simulink model "OFDM_Tx_Rx_Loopback"  (R2020a)
settings: Solver=FixedStepDiscrete  StartTime=0.0  StopTime=inf  RelTol=1e-3
InitFcn:
  | % Set parameters
  | fs = 200e3;
  | 
  | % Load all required variables
  | load('read_addr_data');
  | load('read_addr_cp');
  | load('read_addr_pream');
  | load('read_addr_rx');
  | load('pilot');
  | load('LTSfreq');
  | load('STSfreq');
  | load('LTSread');
  | load('STSread');
  | load('bpsk');
  | load('qpsk');
  | load('qam16');
values from neighbouring files (symbols this model uses):
  bpsk = [0 0 1 1 1 1 0 0 1 0 1 0 ... (48 elements, 48x1)]    [bpsk.mat]
  qam16 = [12 5 10 3 14 8 1 10 8 7 2 13 ... (48 elements, 48x1)]    [qam16.mat]
  qpsk = [1 2 1 2 2 2 3 1 1 3 1 0 ... (48 elements, 48x1)]    [qpsk.mat]
  STSfreq = [0 0 0 0 0 0 0 0 1 0 0 0 ... (64 elements, 1x64)]    [STSfreq.mat]
undefined symbols (not defined in the file or in its folder): data3, LTSfreq, LTSread, pilot, read_addr_cp, read_addr_data, read_addr_pream, read_addr_rx, STSread
libraries: hdlsllib x54, simulink x27, dsphdlxfrm x2, dsphdlsigops x1, dsphdlmathfun x1
(part 3 of 4)

== system OFDM_Tx_Rx_Loopback/OFDMRx/ChannelEstEq/DataArrange/SCReArrange/READ_CTRL ==
  In1 : Inport
  In2 : Inport  Port=2
  Constant : Constant  Value=0  OutDataTypeStr=fixdt(0,7,0)  SampleTime=1/fs
  Switch : Switch  Criteria=u2 ~= 0
  Out1 : Outport  VectorParamsAs1DForOutWhenUnconnected=off
  wires:
  Constant/1 -> Switch/3
  In2/1 -> Switch/2
  In1/1 -> Switch/1
  Switch/1 -> Out1/1

== system OFDM_Tx_Rx_Loopback/OFDMRx/Synchronisation/CoarseTiming/CoarseTimeStrobeGen/LocalSearchCounter ==
  note: Counter starts at 0
  note: Sample counter which is for local serach of X samples
      | after frame starting point. The counter resets
      | after X samples and is only initiated when the frame
      | detection pulse goes HIGH.
  packDetIn : Inport
  Compare To Constant : simulink/Logic and Bit Operations/Compare To Constant  relop===  const=19  OutDataTypeStr=boolean
  Constant : Constant  OutDataTypeStr=boolean  SampleTime=1/fs
  HDL Counter : hdlsllib/Sources/HDL Counter  CountType=Count limited  CountInit=0  CountStep=1  CountMax=19  CountFromType=Initial value  CountFrom=0  CountResetPort=on  CountLoadPort=off  CountEnbPort=on  CountDirPort=off  CountDataType=Unsigned  CountWordLen=8  CountFracLen=0  CountSampTime=1
  NOT : Logic  Operator=NOT  IconShape=distinctive  AllPortsSameDT=off  OutDataTypeStr=boolean
  RsingEdge : Subsystem
  Unit Delay Enabled Resettable Synchronous : hdlsllib/Discrete/Unit Delay Enabled Resettable Synchronous  InitialCondition=0.0  SampleTime=-1
      settings: SourceProductBaseCode=SL
  coutEnb : Outport  VectorParamsAs1DForOutWhenUnconnected=off
  countOut : Outport  Port=2  VectorParamsAs1DForOutWhenUnconnected=off
  wires:
  Unit Delay Enabled Resettable Synchronous/1 -> NOT/1, HDL Counter/2, coutEnb/1
  Compare To Constant/1 -> Unit Delay Enabled Resettable Synchronous/3
  Constant/1 -> Unit Delay Enabled Resettable Synchronous/1
  HDL Counter/1 -> Compare To Constant/1, countOut/1
  RsingEdge/1(Out1) -> Unit Delay Enabled Resettable Synchronous/2
  packDetIn/1 -> RsingEdge/1(In1)
  NOT/1 -> HDL Counter/1

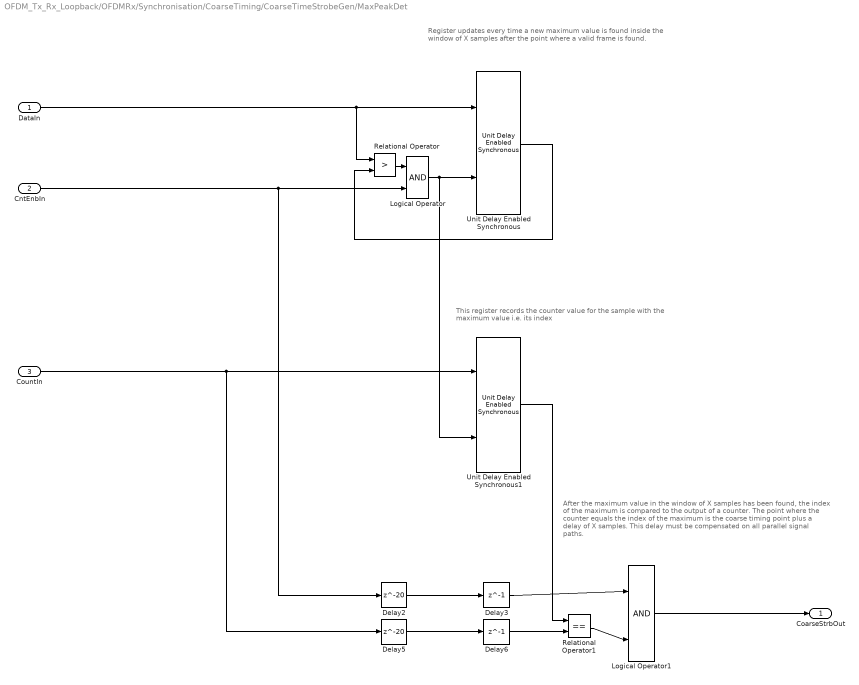
== system OFDM_Tx_Rx_Loopback/OFDMRx/Synchronisation/CoarseTiming/CoarseTimeStrobeGen/MaxPeakDet ==
  note: After the maximum value in the window of X samples has
      | been found, the index of the maximum is compared to the
      | output of a counter. The point where the counter equals the
      | index of the maximum is the coarse timing point plus a delay
      | of X samples. This delay must be compensated on all parallel
      | signal paths.
  note: This register records the counter value for the sample
      | with the maximum value i.e. its index
  note: Register updates every time a new maximum value is
      | found inside the window of X samples after the point where
      | a valid frame is found.
  DataIn : Inport
  CntEnbIn : Inport  Port=2
  CountIn : Inport  Port=3
  Delay2 : Delay  DelayLength=20
  Delay3 : Delay  DelayLength=1
  Delay5 : Delay  DelayLength=20
  Delay6 : Delay  DelayLength=1
  Logical Operator : Logic  IconShape=distinctive  AllPortsSameDT=off  OutDataTypeStr=boolean
  Logical Operator1 : Logic  IconShape=distinctive  AllPortsSameDT=off  OutDataTypeStr=boolean
  Relational Operator : RelationalOperator  Operator=>  OutDataTypeStr=boolean  RndMeth=Nearest
  Relational Operator1 : RelationalOperator  Operator===  OutDataTypeStr=boolean  RndMeth=Nearest
  Unit Delay Enabled Synchronous : hdlsllib/Discrete/Unit Delay Enabled Synchronous  InitialCondition=0.0  SampleTime=-1
      settings: SourceProductBaseCode=SL
  Unit Delay Enabled Synchronous1 : hdlsllib/Discrete/Unit Delay Enabled Synchronous  InitialCondition=0.0  SampleTime=-1
      settings: SourceProductBaseCode=SL
  CoarseStrbOut : Outport  VectorParamsAs1DForOutWhenUnconnected=off
  wires:
  Logical Operator1/1 -> CoarseStrbOut/1
  CountIn/1 -> Delay5/1, Unit Delay Enabled Synchronous1/1
  CntEnbIn/1 -> Delay2/1, Logical Operator/2
  Delay5/1 -> Delay6/1
  Unit Delay Enabled Synchronous/1 -> Relational Operator/2
  Unit Delay Enabled Synchronous1/1 -> Relational Operator1/1
  Relational Operator1/1 -> Logical Operator1/2
  Delay3/1 -> Logical Operator1/1
  Delay2/1 -> Delay3/1
  Relational Operator/1 -> Logical Operator/1
  DataIn/1 -> Unit Delay Enabled Synchronous/1, Relational Operator/1
  Logical Operator/1 -> Unit Delay Enabled Synchronous/2, Unit Delay Enabled Synchronous1/2
  Delay6/1 -> Relational Operator1/2

== system OFDM_Tx_Rx_Loopback/OFDMRx/Synchronisation/ControlSigGen/PreambleValidGen/RisingEdge ==
  ValidIn : Inport
  Delay : Delay  DelayLength=1
  Relational Operator : RelationalOperator  Operator=>  OutDataTypeStr=boolean  RndMeth=Nearest
  Out1 : Outport
  wires:
  Relational Operator/1 -> Out1/1
  Delay/1 -> Relational Operator/2
  ValidIn/1 -> Delay/1, Relational Operator/1

== system OFDM_Tx_Rx_Loopback/OFDMRx/Synchronisation/FineTimingSynch/MatchedFilter/Adder ==
  In1 : Inport
  In2 : Inport  Port=2
  Add : Sum  AccumDataTypeStr=fixdt(1,24,14)
  Delay3 : Delay  DelayLength=1
  Out1 : Outport  VectorParamsAs1DForOutWhenUnconnected=off
  wires:
  In2/1 -> Delay3/1
  In1/1 -> Add/1
  Add/1 -> Out1/1
  Delay3/1 -> Add/2

== system OFDM_Tx_Rx_Loopback/OFDMRx/Synchronisation/FineTimingSynch/MatchedFilter/Adder1 ==
  In1 : Inport
  In2 : Inport  Port=2
  Add : Sum  AccumDataTypeStr=fixdt(1,24,14)
  Delay3 : Delay  DelayLength=1
  Out1 : Outport  VectorParamsAs1DForOutWhenUnconnected=off
  wires:
  Delay3/1 -> Add/2
  Add/1 -> Out1/1
  In1/1 -> Add/1
  In2/1 -> Delay3/1

== system OFDM_Tx_Rx_Loopback/OFDMRx/Synchronisation/FineTimingSynch/MatchedFilter/Adder10 ==
  In1 : Inport
  In2 : Inport  Port=2
  Add : Sum  AccumDataTypeStr=fixdt(1,24,14)
  Delay3 : Delay  DelayLength=1
  Out1 : Outport  VectorParamsAs1DForOutWhenUnconnected=off
  wires:
  In2/1 -> Delay3/1
  In1/1 -> Add/1
  Add/1 -> Out1/1
  Delay3/1 -> Add/2

== system OFDM_Tx_Rx_Loopback/OFDMRx/Synchronisation/FineTimingSynch/MatchedFilter/Adder11 ==
  In1 : Inport
  In2 : Inport  Port=2
  Add : Sum  AccumDataTypeStr=fixdt(1,24,14)
  Delay3 : Delay  DelayLength=1
  Out1 : Outport  VectorParamsAs1DForOutWhenUnconnected=off
  wires:
  Delay3/1 -> Add/2
  Add/1 -> Out1/1
  In1/1 -> Add/1
  In2/1 -> Delay3/1

== system OFDM_Tx_Rx_Loopback/OFDMRx/Synchronisation/FineTimingSynch/MatchedFilter/Adder12 ==
  In1 : Inport
  In2 : Inport  Port=2
  Add : Sum  AccumDataTypeStr=fixdt(1,24,14)
  Delay3 : Delay  DelayLength=1
  Out1 : Outport  VectorParamsAs1DForOutWhenUnconnected=off
  wires:
  In2/1 -> Delay3/1
  In1/1 -> Add/1
  Add/1 -> Out1/1
  Delay3/1 -> Add/2

== system OFDM_Tx_Rx_Loopback/OFDMRx/Synchronisation/FineTimingSynch/MatchedFilter/Adder13 ==
  In1 : Inport
  In2 : Inport  Port=2
  Add : Sum  AccumDataTypeStr=fixdt(1,24,14)
  Delay3 : Delay  DelayLength=1
  Out1 : Outport  VectorParamsAs1DForOutWhenUnconnected=off
  wires:
  Delay3/1 -> Add/2
  Add/1 -> Out1/1
  In1/1 -> Add/1
  In2/1 -> Delay3/1

== system OFDM_Tx_Rx_Loopback/OFDMRx/Synchronisation/FineTimingSynch/MatchedFilter/Adder14 ==
  In1 : Inport
  In2 : Inport  Port=2
  Add : Sum  AccumDataTypeStr=fixdt(1,24,14)
  Delay3 : Delay  DelayLength=1
  Out1 : Outport  VectorParamsAs1DForOutWhenUnconnected=off
  wires:
  In2/1 -> Delay3/1
  In1/1 -> Add/1
  Add/1 -> Out1/1
  Delay3/1 -> Add/2

== system OFDM_Tx_Rx_Loopback/OFDMRx/Synchronisation/FineTimingSynch/MatchedFilter/Adder15 ==
  In1 : Inport
  In2 : Inport  Port=2
  Add : Sum  AccumDataTypeStr=fixdt(1,24,14)
  Delay3 : Delay  DelayLength=1
  Out1 : Outport  VectorParamsAs1DForOutWhenUnconnected=off
  wires:
  Delay3/1 -> Add/2
  Add/1 -> Out1/1
  In1/1 -> Add/1
  In2/1 -> Delay3/1

== system OFDM_Tx_Rx_Loopback/OFDMRx/Synchronisation/FineTimingSynch/MatchedFilter/Adder16 ==
  In1 : Inport
  In2 : Inport  Port=2
  Add : Sum  AccumDataTypeStr=fixdt(1,24,14)
  Delay3 : Delay  DelayLength=1
  Out1 : Outport  VectorParamsAs1DForOutWhenUnconnected=off
  wires:
  In2/1 -> Delay3/1
  In1/1 -> Add/1
  Add/1 -> Out1/1
  Delay3/1 -> Add/2

== system OFDM_Tx_Rx_Loopback/OFDMRx/Synchronisation/FineTimingSynch/MatchedFilter/Adder17 ==
  In1 : Inport
  In2 : Inport  Port=2
  Add : Sum  AccumDataTypeStr=fixdt(1,24,14)
  Delay3 : Delay  DelayLength=1
  Out1 : Outport  VectorParamsAs1DForOutWhenUnconnected=off
  wires:
  Delay3/1 -> Add/2
  Add/1 -> Out1/1
  In1/1 -> Add/1
  In2/1 -> Delay3/1

== system OFDM_Tx_Rx_Loopback/OFDMRx/Synchronisation/FineTimingSynch/MatchedFilter/Adder18 ==
  In1 : Inport
  In2 : Inport  Port=2
  Add : Sum  AccumDataTypeStr=fixdt(1,24,14)
  Delay3 : Delay  DelayLength=1
  Out1 : Outport  VectorParamsAs1DForOutWhenUnconnected=off
  wires:
  In2/1 -> Delay3/1
  In1/1 -> Add/1
  Add/1 -> Out1/1
  Delay3/1 -> Add/2

== system OFDM_Tx_Rx_Loopback/OFDMRx/Synchronisation/FineTimingSynch/MatchedFilter/Adder19 ==
  In1 : Inport
  In2 : Inport  Port=2
  Add : Sum  AccumDataTypeStr=fixdt(1,24,14)
  Delay3 : Delay  DelayLength=1
  Out1 : Outport  VectorParamsAs1DForOutWhenUnconnected=off
  wires:
  In2/1 -> Delay3/1
  In1/1 -> Add/1
  Add/1 -> Out1/1
  Delay3/1 -> Add/2

== system OFDM_Tx_Rx_Loopback/OFDMRx/Synchronisation/FineTimingSynch/MatchedFilter/Adder2 ==
  In1 : Inport
  In2 : Inport  Port=2
  Add : Sum  AccumDataTypeStr=fixdt(1,24,14)
  Delay3 : Delay  DelayLength=1
  Out1 : Outport  VectorParamsAs1DForOutWhenUnconnected=off
  wires:
  In2/1 -> Delay3/1
  In1/1 -> Add/1
  Add/1 -> Out1/1
  Delay3/1 -> Add/2

== system OFDM_Tx_Rx_Loopback/OFDMRx/Synchronisation/FineTimingSynch/MatchedFilter/Adder20 ==
  In1 : Inport
  In2 : Inport  Port=2
  Add : Sum  AccumDataTypeStr=fixdt(1,24,14)
  Delay3 : Delay  DelayLength=1
  Out1 : Outport  VectorParamsAs1DForOutWhenUnconnected=off
  wires:
  In2/1 -> Delay3/1
  In1/1 -> Add/1
  Add/1 -> Out1/1
  Delay3/1 -> Add/2

== system OFDM_Tx_Rx_Loopback/OFDMRx/Synchronisation/FineTimingSynch/MatchedFilter/Adder21 ==
  In1 : Inport
  In2 : Inport  Port=2
  Add : Sum  AccumDataTypeStr=fixdt(1,24,14)
  Delay3 : Delay  DelayLength=1
  Out1 : Outport  VectorParamsAs1DForOutWhenUnconnected=off
  wires:
  In2/1 -> Delay3/1
  In1/1 -> Add/1
  Add/1 -> Out1/1
  Delay3/1 -> Add/2

== system OFDM_Tx_Rx_Loopback/OFDMRx/Synchronisation/FineTimingSynch/MatchedFilter/Adder22 ==
  In1 : Inport
  In2 : Inport  Port=2
  Add : Sum  AccumDataTypeStr=fixdt(1,24,14)
  Delay3 : Delay  DelayLength=1
  Out1 : Outport  VectorParamsAs1DForOutWhenUnconnected=off
  wires:
  In2/1 -> Delay3/1
  In1/1 -> Add/1
  Add/1 -> Out1/1
  Delay3/1 -> Add/2

== system OFDM_Tx_Rx_Loopback/OFDMRx/Synchronisation/FineTimingSynch/MatchedFilter/Adder23 ==
  In1 : Inport
  In2 : Inport  Port=2
  Add : Sum  AccumDataTypeStr=fixdt(1,24,14)
  Delay3 : Delay  DelayLength=1
  Out1 : Outport  VectorParamsAs1DForOutWhenUnconnected=off
  wires:
  In2/1 -> Delay3/1
  In1/1 -> Add/1
  Add/1 -> Out1/1
  Delay3/1 -> Add/2

== system OFDM_Tx_Rx_Loopback/OFDMRx/Synchronisation/FineTimingSynch/MatchedFilter/Adder24 ==
  In1 : Inport
  In2 : Inport  Port=2
  Add : Sum  AccumDataTypeStr=fixdt(1,24,14)
  Delay3 : Delay  DelayLength=1
  Out1 : Outport  VectorParamsAs1DForOutWhenUnconnected=off
  wires:
  In2/1 -> Delay3/1
  In1/1 -> Add/1
  Add/1 -> Out1/1
  Delay3/1 -> Add/2

== system OFDM_Tx_Rx_Loopback/OFDMRx/Synchronisation/FineTimingSynch/MatchedFilter/Adder25 ==
  In1 : Inport
  In2 : Inport  Port=2
  Add : Sum  AccumDataTypeStr=fixdt(1,24,14)
  Delay3 : Delay  DelayLength=1
  Out1 : Outport  VectorParamsAs1DForOutWhenUnconnected=off
  wires:
  In2/1 -> Delay3/1
  In1/1 -> Add/1
  Add/1 -> Out1/1
  Delay3/1 -> Add/2

== system OFDM_Tx_Rx_Loopback/OFDMRx/Synchronisation/FineTimingSynch/MatchedFilter/Adder26 ==
  In1 : Inport
  In2 : Inport  Port=2
  Add : Sum  AccumDataTypeStr=fixdt(1,24,14)
  Delay3 : Delay  DelayLength=1
  Out1 : Outport  VectorParamsAs1DForOutWhenUnconnected=off
  wires:
  In2/1 -> Delay3/1
  In1/1 -> Add/1
  Add/1 -> Out1/1
  Delay3/1 -> Add/2

== system OFDM_Tx_Rx_Loopback/OFDMRx/Synchronisation/FineTimingSynch/MatchedFilter/Adder27 ==
  In1 : Inport
  In2 : Inport  Port=2
  Add : Sum  AccumDataTypeStr=fixdt(1,24,14)
  Delay3 : Delay  DelayLength=1
  Out1 : Outport  VectorParamsAs1DForOutWhenUnconnected=off
  wires:
  In2/1 -> Delay3/1
  In1/1 -> Add/1
  Add/1 -> Out1/1
  Delay3/1 -> Add/2

== system OFDM_Tx_Rx_Loopback/OFDMRx/Synchronisation/FineTimingSynch/MatchedFilter/Adder28 ==
  In1 : Inport
  In2 : Inport  Port=2
  Add : Sum
  Delay3 : Delay  DelayLength=1
  Out1 : Outport  VectorParamsAs1DForOutWhenUnconnected=off
  wires:
  In2/1 -> Delay3/1
  In1/1 -> Add/1
  Add/1 -> Out1/1
  Delay3/1 -> Add/2

== system OFDM_Tx_Rx_Loopback/OFDMRx/Synchronisation/FineTimingSynch/MatchedFilter/Adder29 ==
  In1 : Inport
  In2 : Inport  Port=2
  Add : Sum  AccumDataTypeStr=fixdt(1,24,14)
  Delay3 : Delay  DelayLength=1
  Out1 : Outport  VectorParamsAs1DForOutWhenUnconnected=off
  wires:
  In2/1 -> Delay3/1
  In1/1 -> Add/1
  Add/1 -> Out1/1
  Delay3/1 -> Add/2

== system OFDM_Tx_Rx_Loopback/OFDMRx/Synchronisation/FineTimingSynch/MatchedFilter/Adder3 ==
  In1 : Inport
  In2 : Inport  Port=2
  Add : Sum  AccumDataTypeStr=fixdt(1,24,14)
  Delay3 : Delay  DelayLength=1
  Out1 : Outport  VectorParamsAs1DForOutWhenUnconnected=off
  wires:
  Delay3/1 -> Add/2
  Add/1 -> Out1/1
  In1/1 -> Add/1
  In2/1 -> Delay3/1

== system OFDM_Tx_Rx_Loopback/OFDMRx/Synchronisation/FineTimingSynch/MatchedFilter/Adder30 ==
  In1 : Inport
  In2 : Inport  Port=2
  Add : Sum  AccumDataTypeStr=fixdt(1,24,14)
  Delay3 : Delay  DelayLength=1
  Out1 : Outport  VectorParamsAs1DForOutWhenUnconnected=off
  wires:
  In2/1 -> Delay3/1
  In1/1 -> Add/1
  Add/1 -> Out1/1
  Delay3/1 -> Add/2

== system OFDM_Tx_Rx_Loopback/OFDMRx/Synchronisation/FineTimingSynch/MatchedFilter/Adder31 ==
  In1 : Inport
  In2 : Inport  Port=2
  Add : Sum  AccumDataTypeStr=fixdt(1,24,14)
  Delay3 : Delay  DelayLength=1
  Out1 : Outport  VectorParamsAs1DForOutWhenUnconnected=off
  wires:
  In2/1 -> Delay3/1
  In1/1 -> Add/1
  Add/1 -> Out1/1
  Delay3/1 -> Add/2

== system OFDM_Tx_Rx_Loopback/OFDMRx/Synchronisation/FineTimingSynch/MatchedFilter/Adder32 ==
  In1 : Inport
  In2 : Inport  Port=2
  Add : Sum  AccumDataTypeStr=fixdt(1,24,14)
  Delay3 : Delay  DelayLength=1
  Out1 : Outport  VectorParamsAs1DForOutWhenUnconnected=off
  wires:
  In2/1 -> Delay3/1
  In1/1 -> Add/1
  Add/1 -> Out1/1
  Delay3/1 -> Add/2

== system OFDM_Tx_Rx_Loopback/OFDMRx/Synchronisation/FineTimingSynch/MatchedFilter/Adder33 ==
  In1 : Inport
  In2 : Inport  Port=2
  Add : Sum  AccumDataTypeStr=fixdt(1,24,14)
  Delay3 : Delay  DelayLength=1
  Out1 : Outport  VectorParamsAs1DForOutWhenUnconnected=off
  wires:
  In2/1 -> Delay3/1
  In1/1 -> Add/1
  Add/1 -> Out1/1
  Delay3/1 -> Add/2

== system OFDM_Tx_Rx_Loopback/OFDMRx/Synchronisation/FineTimingSynch/MatchedFilter/Adder34 ==
  In1 : Inport
  In2 : Inport  Port=2
  Add : Sum  AccumDataTypeStr=fixdt(1,24,14)
  Delay3 : Delay  DelayLength=1
  Out1 : Outport  VectorParamsAs1DForOutWhenUnconnected=off
  wires:
  In2/1 -> Delay3/1
  In1/1 -> Add/1
  Add/1 -> Out1/1
  Delay3/1 -> Add/2

== system OFDM_Tx_Rx_Loopback/OFDMRx/Synchronisation/FineTimingSynch/MatchedFilter/Adder35 ==
  In1 : Inport
  In2 : Inport  Port=2
  Add : Sum  AccumDataTypeStr=fixdt(1,24,14)
  Delay3 : Delay  DelayLength=1
  Out1 : Outport  VectorParamsAs1DForOutWhenUnconnected=off
  wires:
  In2/1 -> Delay3/1
  In1/1 -> Add/1
  Add/1 -> Out1/1
  Delay3/1 -> Add/2

== system OFDM_Tx_Rx_Loopback/OFDMRx/Synchronisation/FineTimingSynch/MatchedFilter/Adder36 ==
  In1 : Inport
  In2 : Inport  Port=2
  Add : Sum  AccumDataTypeStr=fixdt(1,24,14)
  Delay3 : Delay  DelayLength=1
  Out1 : Outport  VectorParamsAs1DForOutWhenUnconnected=off
  wires:
  In2/1 -> Delay3/1
  In1/1 -> Add/1
  Add/1 -> Out1/1
  Delay3/1 -> Add/2

== system OFDM_Tx_Rx_Loopback/OFDMRx/Synchronisation/FineTimingSynch/MatchedFilter/Adder37 ==
  In1 : Inport
  In2 : Inport  Port=2
  Add : Sum  AccumDataTypeStr=fixdt(1,24,14)
  Delay3 : Delay  DelayLength=1
  Out1 : Outport  VectorParamsAs1DForOutWhenUnconnected=off
  wires:
  In2/1 -> Delay3/1
  In1/1 -> Add/1
  Add/1 -> Out1/1
  Delay3/1 -> Add/2

== system OFDM_Tx_Rx_Loopback/OFDMRx/Synchronisation/FineTimingSynch/MatchedFilter/Adder38 ==
  In1 : Inport
  In2 : Inport  Port=2
  Add : Sum  AccumDataTypeStr=fixdt(1,24,14)
  Delay3 : Delay  DelayLength=1
  Out1 : Outport  VectorParamsAs1DForOutWhenUnconnected=off
  wires:
  In2/1 -> Delay3/1
  In1/1 -> Add/1
  Add/1 -> Out1/1
  Delay3/1 -> Add/2

== system OFDM_Tx_Rx_Loopback/OFDMRx/Synchronisation/FineTimingSynch/MatchedFilter/Adder39 ==
  In1 : Inport
  In2 : Inport  Port=2
  Add : Sum  AccumDataTypeStr=fixdt(1,24,14)
  Delay3 : Delay  DelayLength=1
  Out1 : Outport  VectorParamsAs1DForOutWhenUnconnected=off
  wires:
  In2/1 -> Delay3/1
  In1/1 -> Add/1
  Add/1 -> Out1/1
  Delay3/1 -> Add/2

== system OFDM_Tx_Rx_Loopback/OFDMRx/Synchronisation/FineTimingSynch/MatchedFilter/Adder4 ==
  In1 : Inport
  In2 : Inport  Port=2
  Add : Sum  AccumDataTypeStr=fixdt(1,24,14)
  Delay3 : Delay  DelayLength=1
  Out1 : Outport  VectorParamsAs1DForOutWhenUnconnected=off
  wires:
  In2/1 -> Delay3/1
  In1/1 -> Add/1
  Add/1 -> Out1/1
  Delay3/1 -> Add/2

== system OFDM_Tx_Rx_Loopback/OFDMRx/Synchronisation/FineTimingSynch/MatchedFilter/Adder40 ==
  In1 : Inport
  In2 : Inport  Port=2
  Add : Sum  AccumDataTypeStr=fixdt(1,24,14)
  Delay3 : Delay  DelayLength=1
  Out1 : Outport  VectorParamsAs1DForOutWhenUnconnected=off
  wires:
  In2/1 -> Delay3/1
  In1/1 -> Add/1
  Add/1 -> Out1/1
  Delay3/1 -> Add/2

== system OFDM_Tx_Rx_Loopback/OFDMRx/Synchronisation/FineTimingSynch/MatchedFilter/Adder41 ==
  In1 : Inport
  In2 : Inport  Port=2
  Add : Sum  AccumDataTypeStr=fixdt(1,24,14)
  Delay3 : Delay  DelayLength=1
  Out1 : Outport  VectorParamsAs1DForOutWhenUnconnected=off
  wires:
  In2/1 -> Delay3/1
  In1/1 -> Add/1
  Add/1 -> Out1/1
  Delay3/1 -> Add/2

== system OFDM_Tx_Rx_Loopback/OFDMRx/Synchronisation/FineTimingSynch/MatchedFilter/Adder42 ==
  In1 : Inport
  In2 : Inport  Port=2
  Add : Sum  AccumDataTypeStr=fixdt(1,24,14)
  Delay3 : Delay  DelayLength=1
  Out1 : Outport  VectorParamsAs1DForOutWhenUnconnected=off
  wires:
  In2/1 -> Delay3/1
  In1/1 -> Add/1
  Add/1 -> Out1/1
  Delay3/1 -> Add/2

== system OFDM_Tx_Rx_Loopback/OFDMRx/Synchronisation/FineTimingSynch/MatchedFilter/Adder43 ==
  In1 : Inport
  In2 : Inport  Port=2
  Add : Sum  AccumDataTypeStr=fixdt(1,24,14)
  Delay3 : Delay  DelayLength=1
  Out1 : Outport  VectorParamsAs1DForOutWhenUnconnected=off
  wires:
  In2/1 -> Delay3/1
  In1/1 -> Add/1
  Add/1 -> Out1/1
  Delay3/1 -> Add/2

== system OFDM_Tx_Rx_Loopback/OFDMRx/Synchronisation/FineTimingSynch/MatchedFilter/Adder44 ==
  In1 : Inport
  In2 : Inport  Port=2
  Add : Sum  AccumDataTypeStr=fixdt(1,24,14)
  Delay3 : Delay  DelayLength=1
  Out1 : Outport  VectorParamsAs1DForOutWhenUnconnected=off
  wires:
  In2/1 -> Delay3/1
  In1/1 -> Add/1
  Add/1 -> Out1/1
  Delay3/1 -> Add/2

== system OFDM_Tx_Rx_Loopback/OFDMRx/Synchronisation/FineTimingSynch/MatchedFilter/Adder45 ==
  In1 : Inport
  In2 : Inport  Port=2
  Add : Sum  AccumDataTypeStr=fixdt(1,24,14)
  Delay3 : Delay  DelayLength=1
  Out1 : Outport  VectorParamsAs1DForOutWhenUnconnected=off
  wires:
  In2/1 -> Delay3/1
  In1/1 -> Add/1
  Add/1 -> Out1/1
  Delay3/1 -> Add/2

== system OFDM_Tx_Rx_Loopback/OFDMRx/Synchronisation/FineTimingSynch/MatchedFilter/Adder46 ==
  In1 : Inport
  In2 : Inport  Port=2
  Add : Sum  AccumDataTypeStr=fixdt(1,24,14)
  Delay3 : Delay  DelayLength=1
  Out1 : Outport  VectorParamsAs1DForOutWhenUnconnected=off
  wires:
  In2/1 -> Delay3/1
  In1/1 -> Add/1
  Add/1 -> Out1/1
  Delay3/1 -> Add/2

== system OFDM_Tx_Rx_Loopback/OFDMRx/Synchronisation/FineTimingSynch/MatchedFilter/Adder47 ==
  In1 : Inport
  In2 : Inport  Port=2
  Add : Sum  AccumDataTypeStr=fixdt(1,24,14)
  Delay3 : Delay  DelayLength=1
  Out1 : Outport  VectorParamsAs1DForOutWhenUnconnected=off
  wires:
  In2/1 -> Delay3/1
  In1/1 -> Add/1
  Add/1 -> Out1/1
  Delay3/1 -> Add/2

== system OFDM_Tx_Rx_Loopback/OFDMRx/Synchronisation/FineTimingSynch/MatchedFilter/Adder48 ==
  In1 : Inport
  In2 : Inport  Port=2
  Add : Sum  AccumDataTypeStr=fixdt(1,24,14)
  Delay3 : Delay  DelayLength=1
  Out1 : Outport  VectorParamsAs1DForOutWhenUnconnected=off
  wires:
  In2/1 -> Delay3/1
  In1/1 -> Add/1
  Add/1 -> Out1/1
  Delay3/1 -> Add/2

== system OFDM_Tx_Rx_Loopback/OFDMRx/Synchronisation/FineTimingSynch/MatchedFilter/Adder49 ==
  In1 : Inport
  In2 : Inport  Port=2
  Add : Sum  AccumDataTypeStr=fixdt(1,24,14)
  Delay3 : Delay  DelayLength=1
  Out1 : Outport  VectorParamsAs1DForOutWhenUnconnected=off
  wires:
  In2/1 -> Delay3/1
  In1/1 -> Add/1
  Add/1 -> Out1/1
  Delay3/1 -> Add/2

== system OFDM_Tx_Rx_Loopback/OFDMRx/Synchronisation/FineTimingSynch/MatchedFilter/Adder5 ==
  In1 : Inport
  In2 : Inport  Port=2
  Add : Sum  AccumDataTypeStr=fixdt(1,24,14)
  Delay3 : Delay  DelayLength=1
  Out1 : Outport  VectorParamsAs1DForOutWhenUnconnected=off
  wires:
  Delay3/1 -> Add/2
  Add/1 -> Out1/1
  In1/1 -> Add/1
  In2/1 -> Delay3/1

== system OFDM_Tx_Rx_Loopback/OFDMRx/Synchronisation/FineTimingSynch/MatchedFilter/Adder50 ==
  In1 : Inport
  In2 : Inport  Port=2
  Add : Sum  AccumDataTypeStr=fixdt(1,24,14)
  Delay3 : Delay  DelayLength=1
  Out1 : Outport  VectorParamsAs1DForOutWhenUnconnected=off
  wires:
  In2/1 -> Delay3/1
  In1/1 -> Add/1
  Add/1 -> Out1/1
  Delay3/1 -> Add/2

== system OFDM_Tx_Rx_Loopback/OFDMRx/Synchronisation/FineTimingSynch/MatchedFilter/Adder51 ==
  In1 : Inport
  In2 : Inport  Port=2
  Add : Sum  AccumDataTypeStr=fixdt(1,24,14)
  Delay3 : Delay  DelayLength=1
  Out1 : Outport  VectorParamsAs1DForOutWhenUnconnected=off
  wires:
  In2/1 -> Delay3/1
  In1/1 -> Add/1
  Add/1 -> Out1/1
  Delay3/1 -> Add/2

== system OFDM_Tx_Rx_Loopback/OFDMRx/Synchronisation/FineTimingSynch/MatchedFilter/Adder52 ==
  In1 : Inport
  In2 : Inport  Port=2
  Add : Sum  AccumDataTypeStr=fixdt(1,24,14)
  Delay3 : Delay  DelayLength=1
  Out1 : Outport  VectorParamsAs1DForOutWhenUnconnected=off
  wires:
  In2/1 -> Delay3/1
  In1/1 -> Add/1
  Add/1 -> Out1/1
  Delay3/1 -> Add/2

== system OFDM_Tx_Rx_Loopback/OFDMRx/Synchronisation/FineTimingSynch/MatchedFilter/Adder53 ==
  In1 : Inport
  In2 : Inport  Port=2
  Add : Sum  AccumDataTypeStr=fixdt(1,24,14)
  Delay3 : Delay  DelayLength=1
  Out1 : Outport  VectorParamsAs1DForOutWhenUnconnected=off
  wires:
  In2/1 -> Delay3/1
  In1/1 -> Add/1
  Add/1 -> Out1/1
  Delay3/1 -> Add/2

== system OFDM_Tx_Rx_Loopback/OFDMRx/Synchronisation/FineTimingSynch/MatchedFilter/Adder54 ==
  In1 : Inport
  In2 : Inport  Port=2
  Add : Sum  AccumDataTypeStr=fixdt(1,24,14)
  Delay3 : Delay  DelayLength=1
  Out1 : Outport  VectorParamsAs1DForOutWhenUnconnected=off
  wires:
  In2/1 -> Delay3/1
  In1/1 -> Add/1
  Add/1 -> Out1/1
  Delay3/1 -> Add/2

== system OFDM_Tx_Rx_Loopback/OFDMRx/Synchronisation/FineTimingSynch/MatchedFilter/Adder55 ==
  In1 : Inport
  In2 : Inport  Port=2
  Add : Sum  AccumDataTypeStr=fixdt(1,24,14)
  Delay3 : Delay  DelayLength=1
  Out1 : Outport  VectorParamsAs1DForOutWhenUnconnected=off
  wires:
  In2/1 -> Delay3/1
  In1/1 -> Add/1
  Add/1 -> Out1/1
  Delay3/1 -> Add/2

== system OFDM_Tx_Rx_Loopback/OFDMRx/Synchronisation/FineTimingSynch/MatchedFilter/Adder56 ==
  In1 : Inport
  In2 : Inport  Port=2
  Add : Sum  AccumDataTypeStr=fixdt(1,24,14)
  Delay3 : Delay  DelayLength=1
  Out1 : Outport  VectorParamsAs1DForOutWhenUnconnected=off
  wires:
  In2/1 -> Delay3/1
  In1/1 -> Add/1
  Add/1 -> Out1/1
  Delay3/1 -> Add/2

== system OFDM_Tx_Rx_Loopback/OFDMRx/Synchronisation/FineTimingSynch/MatchedFilter/Adder57 ==
  In1 : Inport
  In2 : Inport  Port=2
  Add : Sum  AccumDataTypeStr=fixdt(1,24,14)
  Delay3 : Delay  DelayLength=1
  Out1 : Outport  VectorParamsAs1DForOutWhenUnconnected=off
  wires:
  In2/1 -> Delay3/1
  In1/1 -> Add/1
  Add/1 -> Out1/1
  Delay3/1 -> Add/2

== system OFDM_Tx_Rx_Loopback/OFDMRx/Synchronisation/FineTimingSynch/MatchedFilter/Adder58 ==
  In1 : Inport
  In2 : Inport  Port=2
  Add : Sum  AccumDataTypeStr=fixdt(1,24,14)
  Delay3 : Delay  DelayLength=1
  Out1 : Outport  VectorParamsAs1DForOutWhenUnconnected=off
  wires:
  In2/1 -> Delay3/1
  In1/1 -> Add/1
  Add/1 -> Out1/1
  Delay3/1 -> Add/2

== system OFDM_Tx_Rx_Loopback/OFDMRx/Synchronisation/FineTimingSynch/MatchedFilter/Adder59 ==
  In1 : Inport
  In2 : Inport  Port=2
  Add : Sum  AccumDataTypeStr=fixdt(1,24,14)
  Delay3 : Delay  DelayLength=1
  Out1 : Outport  VectorParamsAs1DForOutWhenUnconnected=off
  wires:
  In2/1 -> Delay3/1
  In1/1 -> Add/1
  Add/1 -> Out1/1
  Delay3/1 -> Add/2

== system OFDM_Tx_Rx_Loopback/OFDMRx/Synchronisation/FineTimingSynch/MatchedFilter/Adder6 ==
  In1 : Inport
  In2 : Inport  Port=2
  Add : Sum  AccumDataTypeStr=fixdt(1,24,14)
  Delay3 : Delay  DelayLength=1
  Out1 : Outport  VectorParamsAs1DForOutWhenUnconnected=off
  wires:
  In2/1 -> Delay3/1
  In1/1 -> Add/1
  Add/1 -> Out1/1
  Delay3/1 -> Add/2

== system OFDM_Tx_Rx_Loopback/OFDMRx/Synchronisation/FineTimingSynch/MatchedFilter/Adder60 ==
  In1 : Inport
  In2 : Inport  Port=2
  Add : Sum  AccumDataTypeStr=fixdt(1,24,14)
  Delay3 : Delay  DelayLength=1
  Out1 : Outport  VectorParamsAs1DForOutWhenUnconnected=off
  wires:
  In2/1 -> Delay3/1
  In1/1 -> Add/1
  Add/1 -> Out1/1
  Delay3/1 -> Add/2

== system OFDM_Tx_Rx_Loopback/OFDMRx/Synchronisation/FineTimingSynch/MatchedFilter/Adder61 ==
  In1 : Inport
  In2 : Inport  Port=2
  Add : Sum  AccumDataTypeStr=fixdt(1,24,14)
  Delay3 : Delay  DelayLength=1
  Out1 : Outport  VectorParamsAs1DForOutWhenUnconnected=off
  wires:
  In2/1 -> Delay3/1
  In1/1 -> Add/1
  Add/1 -> Out1/1
  Delay3/1 -> Add/2

== system OFDM_Tx_Rx_Loopback/OFDMRx/Synchronisation/FineTimingSynch/MatchedFilter/Adder62 ==
  In1 : Inport
  In2 : Inport  Port=2
  Add : Sum  AccumDataTypeStr=fixdt(1,24,14)
  Delay3 : Delay  DelayLength=1
  Out1 : Outport  VectorParamsAs1DForOutWhenUnconnected=off
  wires:
  In2/1 -> Delay3/1
  In1/1 -> Add/1
  Add/1 -> Out1/1
  Delay3/1 -> Add/2

== system OFDM_Tx_Rx_Loopback/OFDMRx/Synchronisation/FineTimingSynch/MatchedFilter/Adder7 ==
  In1 : Inport
  In2 : Inport  Port=2
  Add : Sum  AccumDataTypeStr=fixdt(1,24,14)
  Delay3 : Delay  DelayLength=1
  Out1 : Outport  VectorParamsAs1DForOutWhenUnconnected=off
  wires:
  Delay3/1 -> Add/2
  Add/1 -> Out1/1
  In1/1 -> Add/1
  In2/1 -> Delay3/1

== system OFDM_Tx_Rx_Loopback/OFDMRx/Synchronisation/FineTimingSynch/MatchedFilter/Adder8 ==
  In1 : Inport
  In2 : Inport  Port=2
  Add : Sum  AccumDataTypeStr=fixdt(1,24,14)
  Delay3 : Delay  DelayLength=1
  Out1 : Outport  VectorParamsAs1DForOutWhenUnconnected=off
  wires:
  In2/1 -> Delay3/1
  In1/1 -> Add/1
  Add/1 -> Out1/1
  Delay3/1 -> Add/2

== system OFDM_Tx_Rx_Loopback/OFDMRx/Synchronisation/FineTimingSynch/MatchedFilter/Adder9 ==
  In1 : Inport
  In2 : Inport  Port=2
  Add : Sum  AccumDataTypeStr=fixdt(1,24,14)
  Delay3 : Delay  DelayLength=1
  Out1 : Outport  VectorParamsAs1DForOutWhenUnconnected=off
  wires:
  Delay3/1 -> Add/2
  Add/1 -> Out1/1
  In1/1 -> Add/1
  In2/1 -> Delay3/1

== system OFDM_Tx_Rx_Loopback/OFDMRx/Synchronisation/FineTimingSynch/MatchedFilter/Subsystem ==
  MatchedIn : Inport
  Add : Sum  OutDataTypeStr=fixdt(1,18,14)
  Add1 : Sum  Inputs=+-  OutDataTypeStr=fixdt(1,18,14)
  Complex to Real-Imag : ComplexToRealImag
  Real-Imag to Complex : RealImagToComplex
  Unary Minus : UnaryMinus
  Out1 : Outport
  wires:
  Real-Imag to Complex/1 -> Out1/1
  MatchedIn/1 -> Complex to Real-Imag/1
  Add1/1 -> Real-Imag to Complex/1
  Complex to Real-Imag/2 -> Add/2, Add1/1
  Complex to Real-Imag/1 -> Add/1, Add1/2
  Add/1 -> Unary Minus/1
  Unary Minus/1 -> Real-Imag to Complex/2

== system OFDM_Tx_Rx_Loopback/OFDMRx/Synchronisation/FineTimingSynch/MatchedFilter/Subsystem1 ==
  MatchedIn : Inport
  Add : Sum  OutDataTypeStr=fixdt(1,18,14)
  Add1 : Sum  Inputs=+-  OutDataTypeStr=fixdt(1,18,14)
  Complex to Real-Imag : ComplexToRealImag
  Real-Imag to Complex : RealImagToComplex
  Out1 : Outport
  wires:
  Complex to Real-Imag/2 -> Add1/1, Add/2
  Add/1 -> Real-Imag to Complex/1
  Add1/1 -> Real-Imag to Complex/2
  Complex to Real-Imag/1 -> Add1/2, Add/1
  MatchedIn/1 -> Complex to Real-Imag/1
  Real-Imag to Complex/1 -> Out1/1

== system OFDM_Tx_Rx_Loopback/OFDMRx/Synchronisation/FineTimingSynch/MatchedFilter/Subsystem10 ==
  MatchedIn : Inport
  Add : Sum  OutDataTypeStr=fixdt(1,18,14)
  Add1 : Sum  Inputs=+-  OutDataTypeStr=fixdt(1,18,14)
  Complex to Real-Imag : ComplexToRealImag
  Real-Imag to Complex : RealImagToComplex
  Unary Minus : UnaryMinus
  Out1 : Outport
  wires:
  Unary Minus/1 -> Real-Imag to Complex/2
  Add/1 -> Unary Minus/1
  Complex to Real-Imag/1 -> Add1/2, Add/1
  Complex to Real-Imag/2 -> Add1/1, Add/2
  Add1/1 -> Real-Imag to Complex/1
  MatchedIn/1 -> Complex to Real-Imag/1
  Real-Imag to Complex/1 -> Out1/1

== system OFDM_Tx_Rx_Loopback/OFDMRx/Synchronisation/FineTimingSynch/MatchedFilter/Subsystem11 ==
  MatchedIn : Inport
  Add : Sum  OutDataTypeStr=fixdt(1,18,14)
  Add1 : Sum  Inputs=+-  OutDataTypeStr=fixdt(1,18,14)
  Complex to Real-Imag : ComplexToRealImag
  Real-Imag to Complex : RealImagToComplex
  Out1 : Outport
  wires:
  Real-Imag to Complex/1 -> Out1/1
  MatchedIn/1 -> Complex to Real-Imag/1
  Complex to Real-Imag/1 -> Add/1, Add1/2
  Add1/1 -> Real-Imag to Complex/2
  Add/1 -> Real-Imag to Complex/1
  Complex to Real-Imag/2 -> Add/2, Add1/1

== system OFDM_Tx_Rx_Loopback/OFDMRx/Synchronisation/FineTimingSynch/MatchedFilter/Subsystem12 ==
  MatchedIn : Inport
  Add : Sum  OutDataTypeStr=fixdt(1,18,14)
  Add1 : Sum  Inputs=+-  OutDataTypeStr=fixdt(1,18,14)
  Complex to Real-Imag : ComplexToRealImag
  Real-Imag to Complex : RealImagToComplex
  Out1 : Outport
  wires:
  Real-Imag to Complex/1 -> Out1/1
  MatchedIn/1 -> Complex to Real-Imag/1
  Complex to Real-Imag/1 -> Add/1, Add1/2
  Add1/1 -> Real-Imag to Complex/2
  Add/1 -> Real-Imag to Complex/1
  Complex to Real-Imag/2 -> Add/2, Add1/1

== system OFDM_Tx_Rx_Loopback/OFDMRx/Synchronisation/FineTimingSynch/MatchedFilter/Subsystem13 ==
  MatchedIn : Inport
  Add : Sum  OutDataTypeStr=fixdt(1,18,14)
  Add1 : Sum  Inputs=+-  OutDataTypeStr=fixdt(1,18,14)
  Complex to Real-Imag : ComplexToRealImag
  Real-Imag to Complex : RealImagToComplex
  Unary Minus : UnaryMinus
  Out1 : Outport
  wires:
  Complex to Real-Imag/2 -> Add1/2, Add/2
  Add/1 -> Unary Minus/1
  Add1/1 -> Real-Imag to Complex/2
  Complex to Real-Imag/1 -> Add1/1, Add/1
  MatchedIn/1 -> Complex to Real-Imag/1
  Real-Imag to Complex/1 -> Out1/1
  Unary Minus/1 -> Real-Imag to Complex/1

== system OFDM_Tx_Rx_Loopback/OFDMRx/Synchronisation/FineTimingSynch/MatchedFilter/Subsystem14 ==
  MatchedIn : Inport
  Add : Sum  OutDataTypeStr=fixdt(1,18,14)
  Add1 : Sum  Inputs=+-  OutDataTypeStr=fixdt(1,18,14)
  Complex to Real-Imag : ComplexToRealImag
  Real-Imag to Complex : RealImagToComplex
  Out1 : Outport
  wires:
  Real-Imag to Complex/1 -> Out1/1
  MatchedIn/1 -> Complex to Real-Imag/1
  Complex to Real-Imag/1 -> Add/1, Add1/2
  Add1/1 -> Real-Imag to Complex/2
  Add/1 -> Real-Imag to Complex/1
  Complex to Real-Imag/2 -> Add/2, Add1/1

== system OFDM_Tx_Rx_Loopback/OFDMRx/Synchronisation/FineTimingSynch/MatchedFilter/Subsystem15 ==
  MatchedIn : Inport
  Add : Sum  OutDataTypeStr=fixdt(1,18,14)
  Add1 : Sum  Inputs=+-  OutDataTypeStr=fixdt(1,18,14)
  Complex to Real-Imag : ComplexToRealImag
  Real-Imag to Complex : RealImagToComplex
  Out1 : Outport
  wires:
  Real-Imag to Complex/1 -> Out1/1
  MatchedIn/1 -> Complex to Real-Imag/1
  Complex to Real-Imag/1 -> Add/1, Add1/2
  Add1/1 -> Real-Imag to Complex/2
  Add/1 -> Real-Imag to Complex/1
  Complex to Real-Imag/2 -> Add/2, Add1/1

== system OFDM_Tx_Rx_Loopback/OFDMRx/Synchronisation/FineTimingSynch/MatchedFilter/Subsystem16 ==
  MatchedIn : Inport
  Add : Sum  OutDataTypeStr=fixdt(1,18,14)
  Add1 : Sum  Inputs=+-  OutDataTypeStr=fixdt(1,18,14)
  Complex to Real-Imag : ComplexToRealImag
  Real-Imag to Complex : RealImagToComplex
  Out1 : Outport
  wires:
  Add/1 -> Real-Imag to Complex/2
  Add1/1 -> Real-Imag to Complex/1
  Complex to Real-Imag/2 -> Add/2, Add1/2
  Complex to Real-Imag/1 -> Add/1, Add1/1
  MatchedIn/1 -> Complex to Real-Imag/1
  Real-Imag to Complex/1 -> Out1/1

== system OFDM_Tx_Rx_Loopback/OFDMRx/Synchronisation/FineTimingSynch/MatchedFilter/Subsystem17 ==
  MatchedIn : Inport
  Add : Sum  OutDataTypeStr=fixdt(1,18,14)
  Add1 : Sum  Inputs=+-  OutDataTypeStr=fixdt(1,18,14)
  Complex to Real-Imag : ComplexToRealImag
  Real-Imag to Complex : RealImagToComplex
  Unary Minus : UnaryMinus
  Out1 : Outport
  wires:
  Unary Minus/1 -> Real-Imag to Complex/1
  Real-Imag to Complex/1 -> Out1/1
  MatchedIn/1 -> Complex to Real-Imag/1
  Complex to Real-Imag/1 -> Add/1, Add1/1
  Add1/1 -> Real-Imag to Complex/2
  Add/1 -> Unary Minus/1
  Complex to Real-Imag/2 -> Add/2, Add1/2

== system OFDM_Tx_Rx_Loopback/OFDMRx/Synchronisation/FineTimingSynch/MatchedFilter/Subsystem18 ==
  MatchedIn : Inport
  Add : Sum  OutDataTypeStr=fixdt(1,18,14)
  Add1 : Sum  Inputs=+-  OutDataTypeStr=fixdt(1,18,14)
  Complex to Real-Imag : ComplexToRealImag
  Real-Imag to Complex : RealImagToComplex
  Unary Minus : UnaryMinus
  Out1 : Outport
  wires:
  Unary Minus/1 -> Real-Imag to Complex/1
  Real-Imag to Complex/1 -> Out1/1
  MatchedIn/1 -> Complex to Real-Imag/1
  Complex to Real-Imag/1 -> Add/1, Add1/1
  Add1/1 -> Real-Imag to Complex/2
  Add/1 -> Unary Minus/1
  Complex to Real-Imag/2 -> Add/2, Add1/2

== system OFDM_Tx_Rx_Loopback/OFDMRx/Synchronisation/FineTimingSynch/MatchedFilter/Subsystem19 ==
  MatchedIn : Inport
  Add : Sum  OutDataTypeStr=fixdt(1,18,14)
  Add1 : Sum  Inputs=+-  OutDataTypeStr=fixdt(1,18,14)
  Complex to Real-Imag : ComplexToRealImag
  Real-Imag to Complex : RealImagToComplex
  Out1 : Outport
  wires:
  Add/1 -> Real-Imag to Complex/2
  Add1/1 -> Real-Imag to Complex/1
  Complex to Real-Imag/2 -> Add/2, Add1/2
  Complex to Real-Imag/1 -> Add/1, Add1/1
  MatchedIn/1 -> Complex to Real-Imag/1
  Real-Imag to Complex/1 -> Out1/1

== system OFDM_Tx_Rx_Loopback/OFDMRx/Synchronisation/FineTimingSynch/MatchedFilter/Subsystem2 ==
  MatchedIn : Inport
  Add : Sum  OutDataTypeStr=fixdt(1,18,14)
  Add1 : Sum  Inputs=+-  OutDataTypeStr=fixdt(1,18,14)
  Complex to Real-Imag : ComplexToRealImag
  Real-Imag to Complex : RealImagToComplex
  Out1 : Outport
  wires:
  Real-Imag to Complex/1 -> Out1/1
  MatchedIn/1 -> Complex to Real-Imag/1
  Complex to Real-Imag/1 -> Add1/1, Add/1
  Complex to Real-Imag/2 -> Add1/2, Add/2
  Add1/1 -> Real-Imag to Complex/1
  Add/1 -> Real-Imag to Complex/2

== system OFDM_Tx_Rx_Loopback/OFDMRx/Synchronisation/FineTimingSynch/MatchedFilter/Subsystem20 ==
  MatchedIn : Inport
  Add : Sum  OutDataTypeStr=fixdt(1,18,14)
  Add1 : Sum  Inputs=+-  OutDataTypeStr=fixdt(1,18,14)
  Complex to Real-Imag : ComplexToRealImag
  Real-Imag to Complex : RealImagToComplex
  Out1 : Outport
  wires:
  Add/1 -> Real-Imag to Complex/2
  Add1/1 -> Real-Imag to Complex/1
  Complex to Real-Imag/2 -> Add/2, Add1/2
  Complex to Real-Imag/1 -> Add/1, Add1/1
  MatchedIn/1 -> Complex to Real-Imag/1
  Real-Imag to Complex/1 -> Out1/1

== system OFDM_Tx_Rx_Loopback/OFDMRx/Synchronisation/FineTimingSynch/MatchedFilter/Subsystem21 ==
  MatchedIn : Inport
  Add : Sum  OutDataTypeStr=fixdt(1,18,14)
  Add1 : Sum  Inputs=+-  OutDataTypeStr=fixdt(1,18,14)
  Complex to Real-Imag : ComplexToRealImag
  Real-Imag to Complex : RealImagToComplex
  Unary Minus : UnaryMinus
  Out1 : Outport
  wires:
  Unary Minus/1 -> Real-Imag to Complex/1
  Real-Imag to Complex/1 -> Out1/1
  MatchedIn/1 -> Complex to Real-Imag/1
  Complex to Real-Imag/1 -> Add/1, Add1/1
  Add1/1 -> Real-Imag to Complex/2
  Add/1 -> Unary Minus/1
  Complex to Real-Imag/2 -> Add/2, Add1/2

== system OFDM_Tx_Rx_Loopback/OFDMRx/Synchronisation/FineTimingSynch/MatchedFilter/Subsystem22 ==
  MatchedIn : Inport
  Add : Sum  OutDataTypeStr=fixdt(1,18,14)
  Add1 : Sum  Inputs=+-  OutDataTypeStr=fixdt(1,18,14)
  Complex to Real-Imag : ComplexToRealImag
  Real-Imag to Complex : RealImagToComplex
  Unary Minus : UnaryMinus
  Out1 : Outport
  wires:
  Unary Minus/1 -> Real-Imag to Complex/2
  Add/1 -> Unary Minus/1
  Complex to Real-Imag/1 -> Add1/2, Add/1
  Complex to Real-Imag/2 -> Add1/1, Add/2
  Add1/1 -> Real-Imag to Complex/1
  MatchedIn/1 -> Complex to Real-Imag/1
  Real-Imag to Complex/1 -> Out1/1

== system OFDM_Tx_Rx_Loopback/OFDMRx/Synchronisation/FineTimingSynch/MatchedFilter/Subsystem23 ==
  MatchedIn : Inport
  Add : Sum  OutDataTypeStr=fixdt(1,18,14)
  Add1 : Sum  Inputs=+-  OutDataTypeStr=fixdt(1,18,14)
  Complex to Real-Imag : ComplexToRealImag
  Real-Imag to Complex : RealImagToComplex
  Unary Minus : UnaryMinus
  Out1 : Outport
  wires:
  Real-Imag to Complex/1 -> Out1/1
  MatchedIn/1 -> Complex to Real-Imag/1
  Add1/1 -> Real-Imag to Complex/1
  Complex to Real-Imag/2 -> Add/2, Add1/1
  Complex to Real-Imag/1 -> Add/1, Add1/2
  Add/1 -> Unary Minus/1
  Unary Minus/1 -> Real-Imag to Complex/2

== system OFDM_Tx_Rx_Loopback/OFDMRx/Synchronisation/FineTimingSynch/MatchedFilter/Subsystem24 ==
  MatchedIn : Inport
  Add : Sum  OutDataTypeStr=fixdt(1,18,14)
  Add1 : Sum  Inputs=+-  OutDataTypeStr=fixdt(1,18,14)
  Complex to Real-Imag : ComplexToRealImag
  Real-Imag to Complex : RealImagToComplex
  Unary Minus : UnaryMinus
  Out1 : Outport
  wires:
  Unary Minus/1 -> Real-Imag to Complex/2
  Add/1 -> Unary Minus/1
  Complex to Real-Imag/1 -> Add1/2, Add/1
  Complex to Real-Imag/2 -> Add1/1, Add/2
  Add1/1 -> Real-Imag to Complex/1
  MatchedIn/1 -> Complex to Real-Imag/1
  Real-Imag to Complex/1 -> Out1/1

== system OFDM_Tx_Rx_Loopback/OFDMRx/Synchronisation/FineTimingSynch/MatchedFilter/Subsystem25 ==
  MatchedIn : Inport
  Add : Sum  OutDataTypeStr=fixdt(1,18,14)
  Add1 : Sum  Inputs=+-  OutDataTypeStr=fixdt(1,18,14)
  Complex to Real-Imag : ComplexToRealImag
  Real-Imag to Complex : RealImagToComplex
  Unary Minus : UnaryMinus
  Out1 : Outport
  wires:
  Real-Imag to Complex/1 -> Out1/1
  MatchedIn/1 -> Complex to Real-Imag/1
  Add1/1 -> Real-Imag to Complex/1
  Complex to Real-Imag/2 -> Add/2, Add1/1
  Complex to Real-Imag/1 -> Add/1, Add1/2
  Add/1 -> Unary Minus/1
  Unary Minus/1 -> Real-Imag to Complex/2

== system OFDM_Tx_Rx_Loopback/OFDMRx/Synchronisation/FineTimingSynch/MatchedFilter/Subsystem26 ==
  MatchedIn : Inport
  Add : Sum  OutDataTypeStr=fixdt(1,18,14)
  Add1 : Sum  Inputs=+-  OutDataTypeStr=fixdt(1,18,14)
  Complex to Real-Imag : ComplexToRealImag
  Real-Imag to Complex : RealImagToComplex
  Out1 : Outport
  wires:
  Real-Imag to Complex/1 -> Out1/1
  MatchedIn/1 -> Complex to Real-Imag/1
  Complex to Real-Imag/1 -> Add/1, Add1/2
  Add1/1 -> Real-Imag to Complex/2
  Add/1 -> Real-Imag to Complex/1
  Complex to Real-Imag/2 -> Add/2, Add1/1

== system OFDM_Tx_Rx_Loopback/OFDMRx/Synchronisation/FineTimingSynch/MatchedFilter/Subsystem27 ==
  MatchedIn : Inport
  Add : Sum  OutDataTypeStr=fixdt(1,18,14)
  Add1 : Sum  Inputs=+-  OutDataTypeStr=fixdt(1,18,14)
  Complex to Real-Imag : ComplexToRealImag
  Real-Imag to Complex : RealImagToComplex
  Unary Minus : UnaryMinus
  Out1 : Outport
  wires:
  Unary Minus/1 -> Real-Imag to Complex/1
  Real-Imag to Complex/1 -> Out1/1
  MatchedIn/1 -> Complex to Real-Imag/1
  Complex to Real-Imag/1 -> Add/1, Add1/1
  Add1/1 -> Real-Imag to Complex/2
  Add/1 -> Unary Minus/1
  Complex to Real-Imag/2 -> Add/2, Add1/2

== system OFDM_Tx_Rx_Loopback/OFDMRx/Synchronisation/FineTimingSynch/MatchedFilter/Subsystem28 ==
  MatchedIn : Inport
  Add : Sum  OutDataTypeStr=fixdt(1,18,14)
  Add1 : Sum  Inputs=+-  OutDataTypeStr=fixdt(1,18,14)
  Complex to Real-Imag : ComplexToRealImag
  Real-Imag to Complex : RealImagToComplex
  Unary Minus : UnaryMinus
  Out1 : Outport
  wires:
  Unary Minus/1 -> Real-Imag to Complex/1
  Real-Imag to Complex/1 -> Out1/1
  MatchedIn/1 -> Complex to Real-Imag/1
  Complex to Real-Imag/1 -> Add/1, Add1/1
  Add1/1 -> Real-Imag to Complex/2
  Add/1 -> Unary Minus/1
  Complex to Real-Imag/2 -> Add/2, Add1/2

== system OFDM_Tx_Rx_Loopback/OFDMRx/Synchronisation/FineTimingSynch/MatchedFilter/Subsystem29 ==
  MatchedIn : Inport
  Add : Sum  OutDataTypeStr=fixdt(1,18,14)
  Add1 : Sum  Inputs=+-  OutDataTypeStr=fixdt(1,18,14)
  Complex to Real-Imag : ComplexToRealImag
  Real-Imag to Complex : RealImagToComplex
  Out1 : Outport
  wires:
  Add/1 -> Real-Imag to Complex/2
  Add1/1 -> Real-Imag to Complex/1
  Complex to Real-Imag/2 -> Add/2, Add1/2
  Complex to Real-Imag/1 -> Add/1, Add1/1
  MatchedIn/1 -> Complex to Real-Imag/1
  Real-Imag to Complex/1 -> Out1/1

== system OFDM_Tx_Rx_Loopback/OFDMRx/Synchronisation/FineTimingSynch/MatchedFilter/Subsystem3 ==
  MatchedIn : Inport
  Add : Sum  OutDataTypeStr=fixdt(1,18,14)
  Add1 : Sum  Inputs=+-  OutDataTypeStr=fixdt(1,18,14)
  Complex to Real-Imag : ComplexToRealImag
  Real-Imag to Complex : RealImagToComplex
  Out1 : Outport
  wires:
  Add/1 -> Real-Imag to Complex/2
  Add1/1 -> Real-Imag to Complex/1
  Complex to Real-Imag/2 -> Add/2, Add1/2
  Complex to Real-Imag/1 -> Add/1, Add1/1
  MatchedIn/1 -> Complex to Real-Imag/1
  Real-Imag to Complex/1 -> Out1/1

== system OFDM_Tx_Rx_Loopback/OFDMRx/Synchronisation/FineTimingSynch/MatchedFilter/Subsystem30 ==
  MatchedIn : Inport
  Add : Sum  OutDataTypeStr=fixdt(1,18,14)
  Add1 : Sum  Inputs=+-  OutDataTypeStr=fixdt(1,18,14)
  Complex to Real-Imag : ComplexToRealImag
  Real-Imag to Complex : RealImagToComplex
  Out1 : Outport
  wires:
  Add/1 -> Real-Imag to Complex/2
  Add1/1 -> Real-Imag to Complex/1
  Complex to Real-Imag/2 -> Add/2, Add1/2
  Complex to Real-Imag/1 -> Add/1, Add1/1
  MatchedIn/1 -> Complex to Real-Imag/1
  Real-Imag to Complex/1 -> Out1/1

== system OFDM_Tx_Rx_Loopback/OFDMRx/Synchronisation/FineTimingSynch/MatchedFilter/Subsystem31 ==
  In1 : Inport
  Complex to Real-Imag : ComplexToRealImag
  Real-Imag to Complex : RealImagToComplex
  Unary Minus : UnaryMinus
  Unary Minus1 : UnaryMinus
  Out1 : Outport
  wires:
  Unary Minus/1 -> Real-Imag to Complex/1
  Real-Imag to Complex/1 -> Out1/1
  Unary Minus1/1 -> Real-Imag to Complex/2
  Complex to Real-Imag/2 -> Unary Minus1/1
  Complex to Real-Imag/1 -> Unary Minus/1
  In1/1 -> Complex to Real-Imag/1

== system OFDM_Tx_Rx_Loopback/OFDMRx/Synchronisation/FineTimingSynch/MatchedFilter/Subsystem32 ==
  MatchedIn : Inport
  Add : Sum  OutDataTypeStr=fixdt(1,18,14)
  Add1 : Sum  Inputs=+-  OutDataTypeStr=fixdt(1,18,14)
  Complex to Real-Imag : ComplexToRealImag
  Real-Imag to Complex : RealImagToComplex
  Out1 : Outport
  wires:
  Real-Imag to Complex/1 -> Out1/1
  MatchedIn/1 -> Complex to Real-Imag/1
  Complex to Real-Imag/1 -> Add/1, Add1/2
  Add1/1 -> Real-Imag to Complex/2
  Add/1 -> Real-Imag to Complex/1
  Complex to Real-Imag/2 -> Add/2, Add1/1

== system OFDM_Tx_Rx_Loopback/OFDMRx/Synchronisation/FineTimingSynch/MatchedFilter/Subsystem33 ==
  MatchedIn : Inport
  Add : Sum  OutDataTypeStr=fixdt(1,18,14)
  Add1 : Sum  Inputs=+-  OutDataTypeStr=fixdt(1,18,14)
  Complex to Real-Imag : ComplexToRealImag
  Real-Imag to Complex : RealImagToComplex
  Out1 : Outport
  wires:
  Real-Imag to Complex/1 -> Out1/1
  MatchedIn/1 -> Complex to Real-Imag/1
  Complex to Real-Imag/1 -> Add/1, Add1/2
  Add1/1 -> Real-Imag to Complex/2
  Add/1 -> Real-Imag to Complex/1
  Complex to Real-Imag/2 -> Add/2, Add1/1

== system OFDM_Tx_Rx_Loopback/OFDMRx/Synchronisation/FineTimingSynch/MatchedFilter/Subsystem34 ==
  MatchedIn : Inport
  Add : Sum  OutDataTypeStr=fixdt(1,18,14)
  Add1 : Sum  Inputs=+-  OutDataTypeStr=fixdt(1,18,14)
  Complex to Real-Imag : ComplexToRealImag
  Real-Imag to Complex : RealImagToComplex
  Unary Minus : UnaryMinus
  Out1 : Outport
  wires:
  Unary Minus/1 -> Real-Imag to Complex/2
  Add/1 -> Unary Minus/1
  Complex to Real-Imag/1 -> Add1/2, Add/1
  Complex to Real-Imag/2 -> Add1/1, Add/2
  Add1/1 -> Real-Imag to Complex/1
  MatchedIn/1 -> Complex to Real-Imag/1
  Real-Imag to Complex/1 -> Out1/1

== system OFDM_Tx_Rx_Loopback/OFDMRx/Synchronisation/FineTimingSynch/MatchedFilter/Subsystem35 ==
  MatchedIn : Inport
  Add : Sum  OutDataTypeStr=fixdt(1,18,14)
  Add1 : Sum  Inputs=+-  OutDataTypeStr=fixdt(1,18,14)
  Complex to Real-Imag : ComplexToRealImag
  Real-Imag to Complex : RealImagToComplex
  Unary Minus : UnaryMinus
  Out1 : Outport
  wires:
  Unary Minus/1 -> Real-Imag to Complex/2
  Add/1 -> Unary Minus/1
  Complex to Real-Imag/1 -> Add1/2, Add/1
  Complex to Real-Imag/2 -> Add1/1, Add/2
  Add1/1 -> Real-Imag to Complex/1
  MatchedIn/1 -> Complex to Real-Imag/1
  Real-Imag to Complex/1 -> Out1/1

== system OFDM_Tx_Rx_Loopback/OFDMRx/Synchronisation/FineTimingSynch/MatchedFilter/Subsystem36 ==
  MatchedIn : Inport
  Add : Sum  OutDataTypeStr=fixdt(1,18,14)
  Add1 : Sum  Inputs=+-  OutDataTypeStr=fixdt(1,18,14)
  Complex to Real-Imag : ComplexToRealImag
  Real-Imag to Complex : RealImagToComplex
  Out1 : Outport
  wires:
  Add/1 -> Real-Imag to Complex/2
  Add1/1 -> Real-Imag to Complex/1
  Complex to Real-Imag/2 -> Add/2, Add1/2
  Complex to Real-Imag/1 -> Add/1, Add1/1
  MatchedIn/1 -> Complex to Real-Imag/1
  Real-Imag to Complex/1 -> Out1/1

== system OFDM_Tx_Rx_Loopback/OFDMRx/Synchronisation/FineTimingSynch/MatchedFilter/Subsystem37 ==
  MatchedIn : Inport
  Add : Sum  OutDataTypeStr=fixdt(1,18,14)
  Add1 : Sum  Inputs=+-  OutDataTypeStr=fixdt(1,18,14)
  Complex to Real-Imag : ComplexToRealImag
  Real-Imag to Complex : RealImagToComplex
  Unary Minus : UnaryMinus
  Out1 : Outport
  wires:
  Unary Minus/1 -> Real-Imag to Complex/1
  Real-Imag to Complex/1 -> Out1/1
  MatchedIn/1 -> Complex to Real-Imag/1
  Complex to Real-Imag/1 -> Add/1, Add1/1
  Add1/1 -> Real-Imag to Complex/2
  Add/1 -> Unary Minus/1
  Complex to Real-Imag/2 -> Add/2, Add1/2

== system OFDM_Tx_Rx_Loopback/OFDMRx/Synchronisation/FineTimingSynch/MatchedFilter/Subsystem38 ==
  MatchedIn : Inport
  Add : Sum  OutDataTypeStr=fixdt(1,18,14)
  Add1 : Sum  Inputs=+-  OutDataTypeStr=fixdt(1,18,14)
  Complex to Real-Imag : ComplexToRealImag
  Real-Imag to Complex : RealImagToComplex
  Unary Minus : UnaryMinus
  Out1 : Outport
  wires:
  Unary Minus/1 -> Real-Imag to Complex/1
  Real-Imag to Complex/1 -> Out1/1
  MatchedIn/1 -> Complex to Real-Imag/1
  Complex to Real-Imag/1 -> Add/1, Add1/1
  Add1/1 -> Real-Imag to Complex/2
  Add/1 -> Unary Minus/1
  Complex to Real-Imag/2 -> Add/2, Add1/2

== system OFDM_Tx_Rx_Loopback/OFDMRx/Synchronisation/FineTimingSynch/MatchedFilter/Subsystem39 ==
  MatchedIn : Inport
  Add : Sum  OutDataTypeStr=fixdt(1,18,14)
  Add1 : Sum  Inputs=+-  OutDataTypeStr=fixdt(1,18,14)
  Complex to Real-Imag : ComplexToRealImag
  Real-Imag to Complex : RealImagToComplex
  Unary Minus : UnaryMinus
  Out1 : Outport
  wires:
  Unary Minus/1 -> Real-Imag to Complex/1
  Real-Imag to Complex/1 -> Out1/1
  MatchedIn/1 -> Complex to Real-Imag/1
  Complex to Real-Imag/1 -> Add/1, Add1/1
  Add1/1 -> Real-Imag to Complex/2
  Add/1 -> Unary Minus/1
  Complex to Real-Imag/2 -> Add/2, Add1/2

== system OFDM_Tx_Rx_Loopback/OFDMRx/Synchronisation/FineTimingSynch/MatchedFilter/Subsystem4 ==
  MatchedIn : Inport
  Add : Sum  OutDataTypeStr=fixdt(1,18,14)
  Add1 : Sum  Inputs=+-  OutDataTypeStr=fixdt(1,18,14)
  Complex to Real-Imag : ComplexToRealImag
  Real-Imag to Complex : RealImagToComplex
  Out1 : Outport
  wires:
  Real-Imag to Complex/1 -> Out1/1
  MatchedIn/1 -> Complex to Real-Imag/1
  Complex to Real-Imag/1 -> Add/1, Add1/2
  Add1/1 -> Real-Imag to Complex/2
  Add/1 -> Real-Imag to Complex/1
  Complex to Real-Imag/2 -> Add/2, Add1/1

== system OFDM_Tx_Rx_Loopback/OFDMRx/Synchronisation/FineTimingSynch/MatchedFilter/Subsystem40 ==
  MatchedIn : Inport
  Add : Sum  OutDataTypeStr=fixdt(1,18,14)
  Add1 : Sum  Inputs=+-  OutDataTypeStr=fixdt(1,18,14)
  Complex to Real-Imag : ComplexToRealImag
  Real-Imag to Complex : RealImagToComplex
  Unary Minus : UnaryMinus
  Out1 : Outport
  wires:
  Complex to Real-Imag/2 -> Add1/2, Add/2
  Add/1 -> Unary Minus/1
  Add1/1 -> Real-Imag to Complex/2
  Complex to Real-Imag/1 -> Add1/1, Add/1
  MatchedIn/1 -> Complex to Real-Imag/1
  Real-Imag to Complex/1 -> Out1/1
  Unary Minus/1 -> Real-Imag to Complex/1

== system OFDM_Tx_Rx_Loopback/OFDMRx/Synchronisation/FineTimingSynch/MatchedFilter/Subsystem41 ==
  MatchedIn : Inport
  Add : Sum  OutDataTypeStr=fixdt(1,18,14)
  Add1 : Sum  Inputs=+-  OutDataTypeStr=fixdt(1,18,14)
  Complex to Real-Imag : ComplexToRealImag
  Real-Imag to Complex : RealImagToComplex
  Unary Minus : UnaryMinus
  Out1 : Outport
  wires:
  Unary Minus/1 -> Real-Imag to Complex/2
  Add/1 -> Unary Minus/1
  Complex to Real-Imag/1 -> Add1/2, Add/1
  Complex to Real-Imag/2 -> Add1/1, Add/2
  Add1/1 -> Real-Imag to Complex/1
  MatchedIn/1 -> Complex to Real-Imag/1
  Real-Imag to Complex/1 -> Out1/1
